simulink subsystem "Gearbox"  (R2020a)
settings: Solver=VariableStepAuto  StartTime=0.0  StopTime=10.0  RelTol=1e-3
libraries: fl_lib x3, sdl_lib x2
settings Model: Creator=Tyler  LastModifiedBy=Tyler

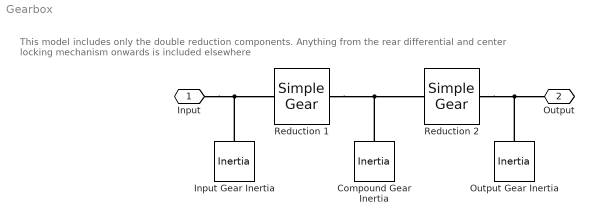
== system Gearbox ==
  note: This model includes only the double reduction components. Anything from the rear differential and center locking mechanism onwards is included elsewhere
  Compound Gear Inertia : fl_lib/Mechanical/Rotational Elements/Inertia  inertia=.00058 kg*m^2  w_specify=off  w_priority=High  w=0 rad/s  w_nominal_specify=off  w_nominal_unit=rad/s  w_nominal_value=1  t_specify=off  t_priority=None  t=0 N*m  t_nominal_specify=off  t_nominal_unit=N*m  t_nominal_value=1
  Input Gear Inertia : fl_lib/Mechanical/Rotational Elements/Inertia  inertia=0.00006 kg*m^2  w_specify=off  w_priority=High  w=0 rad/s  w_nominal_specify=off  w_nominal_unit=rad/s  w_nominal_value=1  t_specify=off  t_priority=None  t=0 N*m  t_nominal_specify=off  t_nominal_unit=N*m  t_nominal_value=1
  Output Gear Inertia : fl_lib/Mechanical/Rotational Elements/Inertia  inertia=.00149 kg*m^2  w_specify=off  w_priority=High  w=0 rad/s  w_nominal_specify=off  w_nominal_unit=rad/s  w_nominal_value=1  t_specify=off  t_priority=None  t=0 N*m  t_nominal_specify=off  t_nominal_unit=N*m  t_nominal_value=1
  Reduction 1 : sdl_lib/Gears/Simple Gear  ratio=48/17  rotation_direction=2  friction_model=sdl.enum.gear_efficiencies_load.constant  T_noload=0.1 N*m  T_nom=5 N*m  efficiency_nom=0.8  efficiency=.95  mu_visc=[0, 0] N*m/(rad/s)  w_thr=0.01 rad/s  pwr_thr=0.001 W  enable_faults=simscape.enum.onoff.off  efficiency_fault=0.05  external_fault=simscape.enum.onoff.off  temporal_fault=simscape.enum.onoff.off  fault_time=5 s  fault_angles=pi / 12 rad  report_fault=1  temperature_TLU=[280, 300, 320] K  load_TLU=[1, 5, 10] N*m  efficiency_TLU=[.95, .9, .85]  efficiency_TLU2=[.85, .8, .75; .95, .9, .85; .85, .8, .7]  thermal_mass=50 J/K  T_init=300 K
  Reduction 2 : sdl_lib/Gears/Simple Gear  ratio=48/17  rotation_direction=2  friction_model=sdl.enum.gear_efficiencies_load.constant  T_noload=0.1 N*m  T_nom=5 N*m  efficiency_nom=0.8  efficiency=.95  mu_visc=[0, 0] N*m/(rad/s)  w_thr=0.01 rad/s  pwr_thr=0.001 W  enable_faults=simscape.enum.onoff.off  efficiency_fault=0.05  external_fault=simscape.enum.onoff.off  temporal_fault=simscape.enum.onoff.off  fault_time=5 s  fault_angles=pi / 12 rad  report_fault=1  temperature_TLU=[280, 300, 320] K  load_TLU=[1, 5, 10] N*m  efficiency_TLU=[.95, .9, .85]  efficiency_TLU2=[.85, .8, .75; .95, .9, .85; .85, .8, .7]  thermal_mass=50 J/K  T_init=300 K
  Input : PMIOPort  Side=Left
  Output : PMIOPort  Port=2  Side=Right
  connections:
  Input Gear Inertia/LConn1 -- Input/RConn1 -- Reduction 1/LConn1
  Compound Gear Inertia/LConn1 -- Reduction 1/RConn1 -- Reduction 2/LConn1
  Output Gear Inertia/LConn1 -- Reduction 2/RConn1 -- Output/RConn1
